simulink model "ExtraCredit"  (R2016a)
settings: Solver=VariableStepAuto  StartTime=0.0  StopTime=10.0  RelTol=1e-3
libraries: hdlsllib x17
(part 2 of 2)

== system ExtraCredit/Subsystem/Subsystem/MultiBlock44 ==
  SumIn : Inport
  Cin : Inport  Port=2
  B : Inport  Port=3
  A : Inport  Port=4
  AND : Logic  IconShape=distinctive  AllPortsSameDT=off  OutDataTypeStr=boolean
  AND1 : Logic  IconShape=distinctive  AllPortsSameDT=off  OutDataTypeStr=boolean
  AND2 : Logic  IconShape=distinctive  AllPortsSameDT=off  OutDataTypeStr=boolean
  "OR " : Logic  Operator=OR  IconShape=distinctive  AllPortsSameDT=off  OutDataTypeStr=boolean
  XOR : Logic  Operator=XOR  IconShape=distinctive  AllPortsSameDT=off  OutDataTypeStr=boolean
  XOR1 : Logic  Operator=XOR  IconShape=distinctive  AllPortsSameDT=off  OutDataTypeStr=boolean
  Sum : Outport
  Carry : Outport  Port=2
  wires:
  SumIn/1 -> XOR1/1, AND/1
  XOR1/1 -> AND1/1, XOR/1
  Cin/1 -> XOR/2, AND1/2
  XOR/1 -> Sum/1
  AND2/1 -> AND/2, XOR1/2
  "OR "/1 -> Carry/1
  AND1/1 -> "OR "/1
  AND/1 -> "OR "/2
  B/1 -> AND2/2
  A/1 -> AND2/1

== system ExtraCredit/Subsystem/Subsystem/MultiBlock45 ==
  SumIn : Inport
  Cin : Inport  Port=2
  B : Inport  Port=3
  A : Inport  Port=4
  AND : Logic  IconShape=distinctive  AllPortsSameDT=off  OutDataTypeStr=boolean
  AND1 : Logic  IconShape=distinctive  AllPortsSameDT=off  OutDataTypeStr=boolean
  AND2 : Logic  IconShape=distinctive  AllPortsSameDT=off  OutDataTypeStr=boolean
  "OR " : Logic  Operator=OR  IconShape=distinctive  AllPortsSameDT=off  OutDataTypeStr=boolean
  XOR : Logic  Operator=XOR  IconShape=distinctive  AllPortsSameDT=off  OutDataTypeStr=boolean
  XOR1 : Logic  Operator=XOR  IconShape=distinctive  AllPortsSameDT=off  OutDataTypeStr=boolean
  Sum : Outport
  Carry : Outport  Port=2
  wires:
  SumIn/1 -> XOR1/1, AND/1
  XOR1/1 -> AND1/1, XOR/1
  Cin/1 -> XOR/2, AND1/2
  XOR/1 -> Sum/1
  AND2/1 -> AND/2, XOR1/2
  "OR "/1 -> Carry/1
  AND1/1 -> "OR "/1
  AND/1 -> "OR "/2
  B/1 -> AND2/2
  A/1 -> AND2/1

== system ExtraCredit/Subsystem/Subsystem/MultiBlock46 ==
  SumIn : Inport
  Cin : Inport  Port=2
  B : Inport  Port=3
  A : Inport  Port=4
  AND : Logic  IconShape=distinctive  AllPortsSameDT=off  OutDataTypeStr=boolean
  AND1 : Logic  IconShape=distinctive  AllPortsSameDT=off  OutDataTypeStr=boolean
  AND2 : Logic  IconShape=distinctive  AllPortsSameDT=off  OutDataTypeStr=boolean
  "OR " : Logic  Operator=OR  IconShape=distinctive  AllPortsSameDT=off  OutDataTypeStr=boolean
  XOR : Logic  Operator=XOR  IconShape=distinctive  AllPortsSameDT=off  OutDataTypeStr=boolean
  XOR1 : Logic  Operator=XOR  IconShape=distinctive  AllPortsSameDT=off  OutDataTypeStr=boolean
  Sum : Outport
  Carry : Outport  Port=2
  wires:
  SumIn/1 -> XOR1/1, AND/1
  XOR1/1 -> AND1/1, XOR/1
  Cin/1 -> XOR/2, AND1/2
  XOR/1 -> Sum/1
  AND2/1 -> AND/2, XOR1/2
  "OR "/1 -> Carry/1
  AND1/1 -> "OR "/1
  AND/1 -> "OR "/2
  B/1 -> AND2/2
  A/1 -> AND2/1

== system ExtraCredit/Subsystem/Subsystem/MultiBlock47 ==
  SumIn : Inport
  Cin : Inport  Port=2
  B : Inport  Port=3
  A : Inport  Port=4
  AND : Logic  IconShape=distinctive  AllPortsSameDT=off  OutDataTypeStr=boolean
  AND1 : Logic  IconShape=distinctive  AllPortsSameDT=off  OutDataTypeStr=boolean
  AND2 : Logic  IconShape=distinctive  AllPortsSameDT=off  OutDataTypeStr=boolean
  "OR " : Logic  Operator=OR  IconShape=distinctive  AllPortsSameDT=off  OutDataTypeStr=boolean
  XOR : Logic  Operator=XOR  IconShape=distinctive  AllPortsSameDT=off  OutDataTypeStr=boolean
  XOR1 : Logic  Operator=XOR  IconShape=distinctive  AllPortsSameDT=off  OutDataTypeStr=boolean
  Sum : Outport
  Carry : Outport  Port=2
  wires:
  SumIn/1 -> XOR1/1, AND/1
  XOR1/1 -> AND1/1, XOR/1
  Cin/1 -> XOR/2, AND1/2
  XOR/1 -> Sum/1
  AND2/1 -> AND/2, XOR1/2
  "OR "/1 -> Carry/1
  AND1/1 -> "OR "/1
  AND/1 -> "OR "/2
  B/1 -> AND2/2
  A/1 -> AND2/1

== system ExtraCredit/Subsystem/Subsystem/MultiBlock48 ==
  SumIn : Inport
  Cin : Inport  Port=2
  B : Inport  Port=3
  A : Inport  Port=4
  AND : Logic  IconShape=distinctive  AllPortsSameDT=off  OutDataTypeStr=boolean
  AND1 : Logic  IconShape=distinctive  AllPortsSameDT=off  OutDataTypeStr=boolean
  AND2 : Logic  IconShape=distinctive  AllPortsSameDT=off  OutDataTypeStr=boolean
  "OR " : Logic  Operator=OR  IconShape=distinctive  AllPortsSameDT=off  OutDataTypeStr=boolean
  XOR : Logic  Operator=XOR  IconShape=distinctive  AllPortsSameDT=off  OutDataTypeStr=boolean
  XOR1 : Logic  Operator=XOR  IconShape=distinctive  AllPortsSameDT=off  OutDataTypeStr=boolean
  Sum : Outport
  Carry : Outport  Port=2
  wires:
  SumIn/1 -> XOR1/1, AND/1
  XOR1/1 -> AND1/1, XOR/1
  Cin/1 -> XOR/2, AND1/2
  XOR/1 -> Sum/1
  AND2/1 -> AND/2, XOR1/2
  "OR "/1 -> Carry/1
  AND1/1 -> "OR "/1
  AND/1 -> "OR "/2
  B/1 -> AND2/2
  A/1 -> AND2/1

== system ExtraCredit/Subsystem/Subsystem/MultiBlock49 ==
  SumIn : Inport
  Cin : Inport  Port=2
  B : Inport  Port=3
  A : Inport  Port=4
  AND : Logic  IconShape=distinctive  AllPortsSameDT=off  OutDataTypeStr=boolean
  AND1 : Logic  IconShape=distinctive  AllPortsSameDT=off  OutDataTypeStr=boolean
  AND2 : Logic  IconShape=distinctive  AllPortsSameDT=off  OutDataTypeStr=boolean
  "OR " : Logic  Operator=OR  IconShape=distinctive  AllPortsSameDT=off  OutDataTypeStr=boolean
  XOR : Logic  Operator=XOR  IconShape=distinctive  AllPortsSameDT=off  OutDataTypeStr=boolean
  XOR1 : Logic  Operator=XOR  IconShape=distinctive  AllPortsSameDT=off  OutDataTypeStr=boolean
  Sum : Outport
  Carry : Outport  Port=2
  wires:
  SumIn/1 -> XOR1/1, AND/1
  XOR1/1 -> AND1/1, XOR/1
  Cin/1 -> XOR/2, AND1/2
  XOR/1 -> Sum/1
  AND2/1 -> AND/2, XOR1/2
  "OR "/1 -> Carry/1
  AND1/1 -> "OR "/1
  AND/1 -> "OR "/2
  B/1 -> AND2/2
  A/1 -> AND2/1

== system ExtraCredit/Subsystem/Subsystem/MultiBlock5 ==
  SumIn : Inport
  Cin : Inport  Port=2
  B : Inport  Port=3
  A : Inport  Port=4
  AND : Logic  IconShape=distinctive  AllPortsSameDT=off  OutDataTypeStr=boolean
  AND1 : Logic  IconShape=distinctive  AllPortsSameDT=off  OutDataTypeStr=boolean
  AND2 : Logic  IconShape=distinctive  AllPortsSameDT=off  OutDataTypeStr=boolean
  "OR " : Logic  Operator=OR  IconShape=distinctive  AllPortsSameDT=off  OutDataTypeStr=boolean
  XOR : Logic  Operator=XOR  IconShape=distinctive  AllPortsSameDT=off  OutDataTypeStr=boolean
  XOR1 : Logic  Operator=XOR  IconShape=distinctive  AllPortsSameDT=off  OutDataTypeStr=boolean
  Sum : Outport
  Carry : Outport  Port=2
  wires:
  SumIn/1 -> XOR1/1, AND/1
  XOR1/1 -> AND1/1, XOR/1
  Cin/1 -> XOR/2, AND1/2
  XOR/1 -> Sum/1
  AND2/1 -> AND/2, XOR1/2
  "OR "/1 -> Carry/1
  AND1/1 -> "OR "/1
  AND/1 -> "OR "/2
  B/1 -> AND2/2
  A/1 -> AND2/1

== system ExtraCredit/Subsystem/Subsystem/MultiBlock50 ==
  SumIn : Inport
  Cin : Inport  Port=2
  B : Inport  Port=3
  A : Inport  Port=4
  AND : Logic  IconShape=distinctive  AllPortsSameDT=off  OutDataTypeStr=boolean
  AND1 : Logic  IconShape=distinctive  AllPortsSameDT=off  OutDataTypeStr=boolean
  AND2 : Logic  IconShape=distinctive  AllPortsSameDT=off  OutDataTypeStr=boolean
  "OR " : Logic  Operator=OR  IconShape=distinctive  AllPortsSameDT=off  OutDataTypeStr=boolean
  XOR : Logic  Operator=XOR  IconShape=distinctive  AllPortsSameDT=off  OutDataTypeStr=boolean
  XOR1 : Logic  Operator=XOR  IconShape=distinctive  AllPortsSameDT=off  OutDataTypeStr=boolean
  Sum : Outport
  Carry : Outport  Port=2
  wires:
  SumIn/1 -> XOR1/1, AND/1
  XOR1/1 -> AND1/1, XOR/1
  Cin/1 -> XOR/2, AND1/2
  XOR/1 -> Sum/1
  AND2/1 -> AND/2, XOR1/2
  "OR "/1 -> Carry/1
  AND1/1 -> "OR "/1
  AND/1 -> "OR "/2
  B/1 -> AND2/2
  A/1 -> AND2/1

== system ExtraCredit/Subsystem/Subsystem/MultiBlock51 ==
  SumIn : Inport
  Cin : Inport  Port=2
  B : Inport  Port=3
  A : Inport  Port=4
  AND : Logic  IconShape=distinctive  AllPortsSameDT=off  OutDataTypeStr=boolean
  AND1 : Logic  IconShape=distinctive  AllPortsSameDT=off  OutDataTypeStr=boolean
  AND2 : Logic  IconShape=distinctive  AllPortsSameDT=off  OutDataTypeStr=boolean
  "OR " : Logic  Operator=OR  IconShape=distinctive  AllPortsSameDT=off  OutDataTypeStr=boolean
  XOR : Logic  Operator=XOR  IconShape=distinctive  AllPortsSameDT=off  OutDataTypeStr=boolean
  XOR1 : Logic  Operator=XOR  IconShape=distinctive  AllPortsSameDT=off  OutDataTypeStr=boolean
  Sum : Outport
  Carry : Outport  Port=2
  wires:
  SumIn/1 -> XOR1/1, AND/1
  XOR1/1 -> AND1/1, XOR/1
  Cin/1 -> XOR/2, AND1/2
  XOR/1 -> Sum/1
  AND2/1 -> AND/2, XOR1/2
  "OR "/1 -> Carry/1
  AND1/1 -> "OR "/1
  AND/1 -> "OR "/2
  B/1 -> AND2/2
  A/1 -> AND2/1

== system ExtraCredit/Subsystem/Subsystem/MultiBlock52 ==
  SumIn : Inport
  Cin : Inport  Port=2
  B : Inport  Port=3
  A : Inport  Port=4
  AND : Logic  IconShape=distinctive  AllPortsSameDT=off  OutDataTypeStr=boolean
  AND1 : Logic  IconShape=distinctive  AllPortsSameDT=off  OutDataTypeStr=boolean
  AND2 : Logic  IconShape=distinctive  AllPortsSameDT=off  OutDataTypeStr=boolean
  "OR " : Logic  Operator=OR  IconShape=distinctive  AllPortsSameDT=off  OutDataTypeStr=boolean
  XOR : Logic  Operator=XOR  IconShape=distinctive  AllPortsSameDT=off  OutDataTypeStr=boolean
  XOR1 : Logic  Operator=XOR  IconShape=distinctive  AllPortsSameDT=off  OutDataTypeStr=boolean
  Sum : Outport
  Carry : Outport  Port=2
  wires:
  SumIn/1 -> XOR1/1, AND/1
  XOR1/1 -> AND1/1, XOR/1
  Cin/1 -> XOR/2, AND1/2
  XOR/1 -> Sum/1
  AND2/1 -> AND/2, XOR1/2
  "OR "/1 -> Carry/1
  AND1/1 -> "OR "/1
  AND/1 -> "OR "/2
  B/1 -> AND2/2
  A/1 -> AND2/1

== system ExtraCredit/Subsystem/Subsystem/MultiBlock53 ==
  SumIn : Inport
  Cin : Inport  Port=2
  B : Inport  Port=3
  A : Inport  Port=4
  AND : Logic  IconShape=distinctive  AllPortsSameDT=off  OutDataTypeStr=boolean
  AND1 : Logic  IconShape=distinctive  AllPortsSameDT=off  OutDataTypeStr=boolean
  AND2 : Logic  IconShape=distinctive  AllPortsSameDT=off  OutDataTypeStr=boolean
  "OR " : Logic  Operator=OR  IconShape=distinctive  AllPortsSameDT=off  OutDataTypeStr=boolean
  XOR : Logic  Operator=XOR  IconShape=distinctive  AllPortsSameDT=off  OutDataTypeStr=boolean
  XOR1 : Logic  Operator=XOR  IconShape=distinctive  AllPortsSameDT=off  OutDataTypeStr=boolean
  Sum : Outport
  Carry : Outport  Port=2
  wires:
  SumIn/1 -> XOR1/1, AND/1
  XOR1/1 -> AND1/1, XOR/1
  Cin/1 -> XOR/2, AND1/2
  XOR/1 -> Sum/1
  AND2/1 -> AND/2, XOR1/2
  "OR "/1 -> Carry/1
  AND1/1 -> "OR "/1
  AND/1 -> "OR "/2
  B/1 -> AND2/2
  A/1 -> AND2/1

== system ExtraCredit/Subsystem/Subsystem/MultiBlock54 ==
  SumIn : Inport
  Cin : Inport  Port=2
  B : Inport  Port=3
  A : Inport  Port=4
  AND : Logic  IconShape=distinctive  AllPortsSameDT=off  OutDataTypeStr=boolean
  AND1 : Logic  IconShape=distinctive  AllPortsSameDT=off  OutDataTypeStr=boolean
  AND2 : Logic  IconShape=distinctive  AllPortsSameDT=off  OutDataTypeStr=boolean
  "OR " : Logic  Operator=OR  IconShape=distinctive  AllPortsSameDT=off  OutDataTypeStr=boolean
  XOR : Logic  Operator=XOR  IconShape=distinctive  AllPortsSameDT=off  OutDataTypeStr=boolean
  XOR1 : Logic  Operator=XOR  IconShape=distinctive  AllPortsSameDT=off  OutDataTypeStr=boolean
  Sum : Outport
  Carry : Outport  Port=2
  wires:
  SumIn/1 -> XOR1/1, AND/1
  XOR1/1 -> AND1/1, XOR/1
  Cin/1 -> XOR/2, AND1/2
  XOR/1 -> Sum/1
  AND2/1 -> AND/2, XOR1/2
  "OR "/1 -> Carry/1
  AND1/1 -> "OR "/1
  AND/1 -> "OR "/2
  B/1 -> AND2/2
  A/1 -> AND2/1

== system ExtraCredit/Subsystem/Subsystem/MultiBlock55 ==
  SumIn : Inport
  Cin : Inport  Port=2
  B : Inport  Port=3
  A : Inport  Port=4
  AND : Logic  IconShape=distinctive  AllPortsSameDT=off  OutDataTypeStr=boolean
  AND1 : Logic  IconShape=distinctive  AllPortsSameDT=off  OutDataTypeStr=boolean
  AND2 : Logic  IconShape=distinctive  AllPortsSameDT=off  OutDataTypeStr=boolean
  "OR " : Logic  Operator=OR  IconShape=distinctive  AllPortsSameDT=off  OutDataTypeStr=boolean
  XOR : Logic  Operator=XOR  IconShape=distinctive  AllPortsSameDT=off  OutDataTypeStr=boolean
  XOR1 : Logic  Operator=XOR  IconShape=distinctive  AllPortsSameDT=off  OutDataTypeStr=boolean
  Sum : Outport
  Carry : Outport  Port=2
  wires:
  SumIn/1 -> XOR1/1, AND/1
  XOR1/1 -> AND1/1, XOR/1
  Cin/1 -> XOR/2, AND1/2
  XOR/1 -> Sum/1
  AND2/1 -> AND/2, XOR1/2
  "OR "/1 -> Carry/1
  AND1/1 -> "OR "/1
  AND/1 -> "OR "/2
  B/1 -> AND2/2
  A/1 -> AND2/1

== system ExtraCredit/Subsystem/Subsystem/MultiBlock56 ==
  SumIn : Inport
  Cin : Inport  Port=2
  B : Inport  Port=3
  A : Inport  Port=4
  AND : Logic  IconShape=distinctive  AllPortsSameDT=off  OutDataTypeStr=boolean
  AND1 : Logic  IconShape=distinctive  AllPortsSameDT=off  OutDataTypeStr=boolean
  AND2 : Logic  IconShape=distinctive  AllPortsSameDT=off  OutDataTypeStr=boolean
  "OR " : Logic  Operator=OR  IconShape=distinctive  AllPortsSameDT=off  OutDataTypeStr=boolean
  XOR : Logic  Operator=XOR  IconShape=distinctive  AllPortsSameDT=off  OutDataTypeStr=boolean
  XOR1 : Logic  Operator=XOR  IconShape=distinctive  AllPortsSameDT=off  OutDataTypeStr=boolean
  Sum : Outport
  Carry : Outport  Port=2
  wires:
  SumIn/1 -> XOR1/1, AND/1
  XOR1/1 -> AND1/1, XOR/1
  Cin/1 -> XOR/2, AND1/2
  XOR/1 -> Sum/1
  AND2/1 -> AND/2, XOR1/2
  "OR "/1 -> Carry/1
  AND1/1 -> "OR "/1
  AND/1 -> "OR "/2
  B/1 -> AND2/2
  A/1 -> AND2/1

== system ExtraCredit/Subsystem/Subsystem/MultiBlock57 ==
  SumIn : Inport
  Cin : Inport  Port=2
  B : Inport  Port=3
  A : Inport  Port=4
  AND : Logic  IconShape=distinctive  AllPortsSameDT=off  OutDataTypeStr=boolean
  AND1 : Logic  IconShape=distinctive  AllPortsSameDT=off  OutDataTypeStr=boolean
  AND2 : Logic  IconShape=distinctive  AllPortsSameDT=off  OutDataTypeStr=boolean
  "OR " : Logic  Operator=OR  IconShape=distinctive  AllPortsSameDT=off  OutDataTypeStr=boolean
  XOR : Logic  Operator=XOR  IconShape=distinctive  AllPortsSameDT=off  OutDataTypeStr=boolean
  XOR1 : Logic  Operator=XOR  IconShape=distinctive  AllPortsSameDT=off  OutDataTypeStr=boolean
  Sum : Outport
  Carry : Outport  Port=2
  wires:
  SumIn/1 -> XOR1/1, AND/1
  XOR1/1 -> AND1/1, XOR/1
  Cin/1 -> XOR/2, AND1/2
  XOR/1 -> Sum/1
  AND2/1 -> AND/2, XOR1/2
  "OR "/1 -> Carry/1
  AND1/1 -> "OR "/1
  AND/1 -> "OR "/2
  B/1 -> AND2/2
  A/1 -> AND2/1

== system ExtraCredit/Subsystem/Subsystem/MultiBlock58 ==
  SumIn : Inport
  Cin : Inport  Port=2
  B : Inport  Port=3
  A : Inport  Port=4
  AND : Logic  IconShape=distinctive  AllPortsSameDT=off  OutDataTypeStr=boolean
  AND1 : Logic  IconShape=distinctive  AllPortsSameDT=off  OutDataTypeStr=boolean
  AND2 : Logic  IconShape=distinctive  AllPortsSameDT=off  OutDataTypeStr=boolean
  "OR " : Logic  Operator=OR  IconShape=distinctive  AllPortsSameDT=off  OutDataTypeStr=boolean
  XOR : Logic  Operator=XOR  IconShape=distinctive  AllPortsSameDT=off  OutDataTypeStr=boolean
  XOR1 : Logic  Operator=XOR  IconShape=distinctive  AllPortsSameDT=off  OutDataTypeStr=boolean
  Sum : Outport
  Carry : Outport  Port=2
  wires:
  SumIn/1 -> XOR1/1, AND/1
  XOR1/1 -> AND1/1, XOR/1
  Cin/1 -> XOR/2, AND1/2
  XOR/1 -> Sum/1
  AND2/1 -> AND/2, XOR1/2
  "OR "/1 -> Carry/1
  AND1/1 -> "OR "/1
  AND/1 -> "OR "/2
  B/1 -> AND2/2
  A/1 -> AND2/1

== system ExtraCredit/Subsystem/Subsystem/MultiBlock59 ==
  SumIn : Inport
  Cin : Inport  Port=2
  B : Inport  Port=3
  A : Inport  Port=4
  AND : Logic  IconShape=distinctive  AllPortsSameDT=off  OutDataTypeStr=boolean
  AND1 : Logic  IconShape=distinctive  AllPortsSameDT=off  OutDataTypeStr=boolean
  AND2 : Logic  IconShape=distinctive  AllPortsSameDT=off  OutDataTypeStr=boolean
  "OR " : Logic  Operator=OR  IconShape=distinctive  AllPortsSameDT=off  OutDataTypeStr=boolean
  XOR : Logic  Operator=XOR  IconShape=distinctive  AllPortsSameDT=off  OutDataTypeStr=boolean
  XOR1 : Logic  Operator=XOR  IconShape=distinctive  AllPortsSameDT=off  OutDataTypeStr=boolean
  Sum : Outport
  Carry : Outport  Port=2
  wires:
  SumIn/1 -> XOR1/1, AND/1
  XOR1/1 -> AND1/1, XOR/1
  Cin/1 -> XOR/2, AND1/2
  XOR/1 -> Sum/1
  AND2/1 -> AND/2, XOR1/2
  "OR "/1 -> Carry/1
  AND1/1 -> "OR "/1
  AND/1 -> "OR "/2
  B/1 -> AND2/2
  A/1 -> AND2/1

== system ExtraCredit/Subsystem/Subsystem/MultiBlock6 ==
  SumIn : Inport
  Cin : Inport  Port=2
  B : Inport  Port=3
  A : Inport  Port=4
  AND : Logic  IconShape=distinctive  AllPortsSameDT=off  OutDataTypeStr=boolean
  AND1 : Logic  IconShape=distinctive  AllPortsSameDT=off  OutDataTypeStr=boolean
  AND2 : Logic  IconShape=distinctive  AllPortsSameDT=off  OutDataTypeStr=boolean
  "OR " : Logic  Operator=OR  IconShape=distinctive  AllPortsSameDT=off  OutDataTypeStr=boolean
  XOR : Logic  Operator=XOR  IconShape=distinctive  AllPortsSameDT=off  OutDataTypeStr=boolean
  XOR1 : Logic  Operator=XOR  IconShape=distinctive  AllPortsSameDT=off  OutDataTypeStr=boolean
  Sum : Outport
  Carry : Outport  Port=2
  wires:
  SumIn/1 -> XOR1/1, AND/1
  XOR1/1 -> AND1/1, XOR/1
  Cin/1 -> XOR/2, AND1/2
  XOR/1 -> Sum/1
  AND2/1 -> AND/2, XOR1/2
  "OR "/1 -> Carry/1
  AND1/1 -> "OR "/1
  AND/1 -> "OR "/2
  B/1 -> AND2/2
  A/1 -> AND2/1

== system ExtraCredit/Subsystem/Subsystem/MultiBlock60 ==
  SumIn : Inport
  Cin : Inport  Port=2
  B : Inport  Port=3
  A : Inport  Port=4
  AND : Logic  IconShape=distinctive  AllPortsSameDT=off  OutDataTypeStr=boolean
  AND1 : Logic  IconShape=distinctive  AllPortsSameDT=off  OutDataTypeStr=boolean
  AND2 : Logic  IconShape=distinctive  AllPortsSameDT=off  OutDataTypeStr=boolean
  "OR " : Logic  Operator=OR  IconShape=distinctive  AllPortsSameDT=off  OutDataTypeStr=boolean
  XOR : Logic  Operator=XOR  IconShape=distinctive  AllPortsSameDT=off  OutDataTypeStr=boolean
  XOR1 : Logic  Operator=XOR  IconShape=distinctive  AllPortsSameDT=off  OutDataTypeStr=boolean
  Sum : Outport
  Carry : Outport  Port=2
  wires:
  SumIn/1 -> XOR1/1, AND/1
  XOR1/1 -> AND1/1, XOR/1
  Cin/1 -> XOR/2, AND1/2
  XOR/1 -> Sum/1
  AND2/1 -> AND/2, XOR1/2
  "OR "/1 -> Carry/1
  AND1/1 -> "OR "/1
  AND/1 -> "OR "/2
  B/1 -> AND2/2
  A/1 -> AND2/1

== system ExtraCredit/Subsystem/Subsystem/MultiBlock61 ==
  SumIn : Inport
  Cin : Inport  Port=2
  B : Inport  Port=3
  A : Inport  Port=4
  AND : Logic  IconShape=distinctive  AllPortsSameDT=off  OutDataTypeStr=boolean
  AND1 : Logic  IconShape=distinctive  AllPortsSameDT=off  OutDataTypeStr=boolean
  AND2 : Logic  IconShape=distinctive  AllPortsSameDT=off  OutDataTypeStr=boolean
  "OR " : Logic  Operator=OR  IconShape=distinctive  AllPortsSameDT=off  OutDataTypeStr=boolean
  XOR : Logic  Operator=XOR  IconShape=distinctive  AllPortsSameDT=off  OutDataTypeStr=boolean
  XOR1 : Logic  Operator=XOR  IconShape=distinctive  AllPortsSameDT=off  OutDataTypeStr=boolean
  Sum : Outport
  Carry : Outport  Port=2
  wires:
  SumIn/1 -> XOR1/1, AND/1
  XOR1/1 -> AND1/1, XOR/1
  Cin/1 -> XOR/2, AND1/2
  XOR/1 -> Sum/1
  AND2/1 -> AND/2, XOR1/2
  "OR "/1 -> Carry/1
  AND1/1 -> "OR "/1
  AND/1 -> "OR "/2
  B/1 -> AND2/2
  A/1 -> AND2/1

== system ExtraCredit/Subsystem/Subsystem/MultiBlock62 ==
  SumIn : Inport
  Cin : Inport  Port=2
  B : Inport  Port=3
  A : Inport  Port=4
  AND : Logic  IconShape=distinctive  AllPortsSameDT=off  OutDataTypeStr=boolean
  AND1 : Logic  IconShape=distinctive  AllPortsSameDT=off  OutDataTypeStr=boolean
  AND2 : Logic  IconShape=distinctive  AllPortsSameDT=off  OutDataTypeStr=boolean
  "OR " : Logic  Operator=OR  IconShape=distinctive  AllPortsSameDT=off  OutDataTypeStr=boolean
  XOR : Logic  Operator=XOR  IconShape=distinctive  AllPortsSameDT=off  OutDataTypeStr=boolean
  XOR1 : Logic  Operator=XOR  IconShape=distinctive  AllPortsSameDT=off  OutDataTypeStr=boolean
  Sum : Outport
  Carry : Outport  Port=2
  wires:
  SumIn/1 -> XOR1/1, AND/1
  XOR1/1 -> AND1/1, XOR/1
  Cin/1 -> XOR/2, AND1/2
  XOR/1 -> Sum/1
  AND2/1 -> AND/2, XOR1/2
  "OR "/1 -> Carry/1
  AND1/1 -> "OR "/1
  AND/1 -> "OR "/2
  B/1 -> AND2/2
  A/1 -> AND2/1

== system ExtraCredit/Subsystem/Subsystem/MultiBlock63 ==
  SumIn : Inport
  Cin : Inport  Port=2
  B : Inport  Port=3
  A : Inport  Port=4
  AND : Logic  IconShape=distinctive  AllPortsSameDT=off  OutDataTypeStr=boolean
  AND1 : Logic  IconShape=distinctive  AllPortsSameDT=off  OutDataTypeStr=boolean
  AND2 : Logic  IconShape=distinctive  AllPortsSameDT=off  OutDataTypeStr=boolean
  "OR " : Logic  Operator=OR  IconShape=distinctive  AllPortsSameDT=off  OutDataTypeStr=boolean
  XOR : Logic  Operator=XOR  IconShape=distinctive  AllPortsSameDT=off  OutDataTypeStr=boolean
  XOR1 : Logic  Operator=XOR  IconShape=distinctive  AllPortsSameDT=off  OutDataTypeStr=boolean
  Sum : Outport
  Carry : Outport  Port=2
  wires:
  SumIn/1 -> XOR1/1, AND/1
  XOR1/1 -> AND1/1, XOR/1
  Cin/1 -> XOR/2, AND1/2
  XOR/1 -> Sum/1
  AND2/1 -> AND/2, XOR1/2
  "OR "/1 -> Carry/1
  AND1/1 -> "OR "/1
  AND/1 -> "OR "/2
  B/1 -> AND2/2
  A/1 -> AND2/1

== system ExtraCredit/Subsystem/Subsystem/MultiBlock7 ==
  SumIn : Inport
  Cin : Inport  Port=2
  B : Inport  Port=3
  A : Inport  Port=4
  AND : Logic  IconShape=distinctive  AllPortsSameDT=off  OutDataTypeStr=boolean
  AND1 : Logic  IconShape=distinctive  AllPortsSameDT=off  OutDataTypeStr=boolean
  AND2 : Logic  IconShape=distinctive  AllPortsSameDT=off  OutDataTypeStr=boolean
  "OR " : Logic  Operator=OR  IconShape=distinctive  AllPortsSameDT=off  OutDataTypeStr=boolean
  XOR : Logic  Operator=XOR  IconShape=distinctive  AllPortsSameDT=off  OutDataTypeStr=boolean
  XOR1 : Logic  Operator=XOR  IconShape=distinctive  AllPortsSameDT=off  OutDataTypeStr=boolean
  Sum : Outport
  Carry : Outport  Port=2
  wires:
  SumIn/1 -> XOR1/1, AND/1
  XOR1/1 -> AND1/1, XOR/1
  Cin/1 -> XOR/2, AND1/2
  XOR/1 -> Sum/1
  AND2/1 -> AND/2, XOR1/2
  "OR "/1 -> Carry/1
  AND1/1 -> "OR "/1
  AND/1 -> "OR "/2
  B/1 -> AND2/2
  A/1 -> AND2/1

== system ExtraCredit/Subsystem/Subsystem/MultiBlock8 ==
  SumIn : Inport
  Cin : Inport  Port=2
  B : Inport  Port=3
  A : Inport  Port=4
  AND : Logic  IconShape=distinctive  AllPortsSameDT=off  OutDataTypeStr=boolean
  AND1 : Logic  IconShape=distinctive  AllPortsSameDT=off  OutDataTypeStr=boolean
  AND2 : Logic  IconShape=distinctive  AllPortsSameDT=off  OutDataTypeStr=boolean
  "OR " : Logic  Operator=OR  IconShape=distinctive  AllPortsSameDT=off  OutDataTypeStr=boolean
  XOR : Logic  Operator=XOR  IconShape=distinctive  AllPortsSameDT=off  OutDataTypeStr=boolean
  XOR1 : Logic  Operator=XOR  IconShape=distinctive  AllPortsSameDT=off  OutDataTypeStr=boolean
  Sum : Outport
  Carry : Outport  Port=2
  wires:
  SumIn/1 -> XOR1/1, AND/1
  XOR1/1 -> AND1/1, XOR/1
  Cin/1 -> XOR/2, AND1/2
  XOR/1 -> Sum/1
  AND2/1 -> AND/2, XOR1/2
  "OR "/1 -> Carry/1
  AND1/1 -> "OR "/1
  AND/1 -> "OR "/2
  B/1 -> AND2/2
  A/1 -> AND2/1

== system ExtraCredit/Subsystem/Subsystem/MultiBlock9 ==
  SumIn : Inport
  Cin : Inport  Port=2
  B : Inport  Port=3
  A : Inport  Port=4
  AND : Logic  IconShape=distinctive  AllPortsSameDT=off  OutDataTypeStr=boolean
  AND1 : Logic  IconShape=distinctive  AllPortsSameDT=off  OutDataTypeStr=boolean
  AND2 : Logic  IconShape=distinctive  AllPortsSameDT=off  OutDataTypeStr=boolean
  "OR " : Logic  Operator=OR  IconShape=distinctive  AllPortsSameDT=off  OutDataTypeStr=boolean
  XOR : Logic  Operator=XOR  IconShape=distinctive  AllPortsSameDT=off  OutDataTypeStr=boolean
  XOR1 : Logic  Operator=XOR  IconShape=distinctive  AllPortsSameDT=off  OutDataTypeStr=boolean
  Sum : Outport
  Carry : Outport  Port=2
  wires:
  SumIn/1 -> XOR1/1, AND/1
  XOR1/1 -> AND1/1, XOR/1
  Cin/1 -> XOR/2, AND1/2
  XOR/1 -> Sum/1
  AND2/1 -> AND/2, XOR1/2
  "OR "/1 -> Carry/1
  AND1/1 -> "OR "/1
  AND/1 -> "OR "/2
  B/1 -> AND2/2
  A/1 -> AND2/1

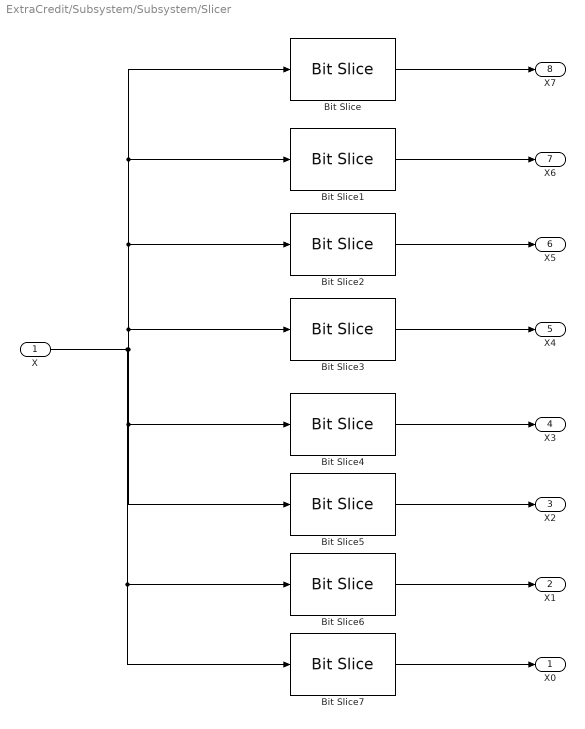
== system ExtraCredit/Subsystem/Subsystem/Slicer ==
  X : Inport  OutDataTypeStr=int8  SampleTime=1
  Bit Slice : hdlsllib/HDL Operations/Bit Slice  lidx=7  ridx=7
  Bit Slice1 : hdlsllib/HDL Operations/Bit Slice  lidx=6  ridx=6
  Bit Slice2 : hdlsllib/HDL Operations/Bit Slice  lidx=5  ridx=5
  Bit Slice3 : hdlsllib/HDL Operations/Bit Slice  lidx=4  ridx=4
  Bit Slice4 : hdlsllib/HDL Operations/Bit Slice  lidx=3  ridx=3
  Bit Slice5 : hdlsllib/HDL Operations/Bit Slice  lidx=2  ridx=2
  Bit Slice6 : hdlsllib/HDL Operations/Bit Slice  lidx=1  ridx=1
  Bit Slice7 : hdlsllib/HDL Operations/Bit Slice  lidx=0  ridx=0
  X0 : Outport
  X1 : Outport  Port=2
  X2 : Outport  Port=3
  X3 : Outport  Port=4
  X4 : Outport  Port=5
  X5 : Outport  Port=6
  X6 : Outport  Port=7
  X7 : Outport  Port=8
  wires:
  Bit Slice7/1 -> X0/1
  Bit Slice6/1 -> X1/1
  Bit Slice3/1 -> X4/1
  Bit Slice/1 -> X7/1
  Bit Slice5/1 -> X2/1
  Bit Slice4/1 -> X3/1
  Bit Slice1/1 -> X6/1
  Bit Slice2/1 -> X5/1
  X/1 -> Bit Slice7/1, Bit Slice6/1, Bit Slice3/1, Bit Slice/1, Bit Slice1/1, Bit Slice2/1, Bit Slice4/1, Bit Slice5/1

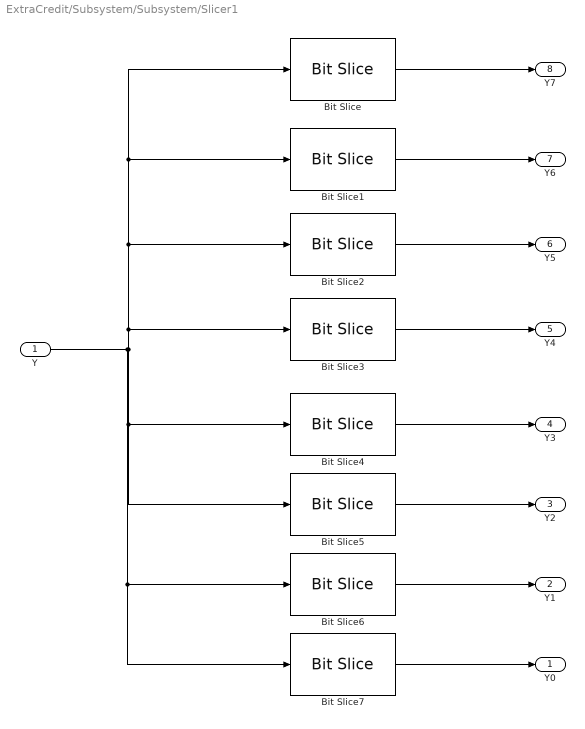
== system ExtraCredit/Subsystem/Subsystem/Slicer1 ==
  Y : Inport  OutDataTypeStr=int8  SampleTime=1
  Bit Slice : hdlsllib/HDL Operations/Bit Slice  lidx=7  ridx=7
  Bit Slice1 : hdlsllib/HDL Operations/Bit Slice  lidx=6  ridx=6
  Bit Slice2 : hdlsllib/HDL Operations/Bit Slice  lidx=5  ridx=5
  Bit Slice3 : hdlsllib/HDL Operations/Bit Slice  lidx=4  ridx=4
  Bit Slice4 : hdlsllib/HDL Operations/Bit Slice  lidx=3  ridx=3
  Bit Slice5 : hdlsllib/HDL Operations/Bit Slice  lidx=2  ridx=2
  Bit Slice6 : hdlsllib/HDL Operations/Bit Slice  lidx=1  ridx=1
  Bit Slice7 : hdlsllib/HDL Operations/Bit Slice  lidx=0  ridx=0
  Y0 : Outport
  Y1 : Outport  Port=2
  Y2 : Outport  Port=3
  Y3 : Outport  Port=4
  Y4 : Outport  Port=5
  Y5 : Outport  Port=6
  Y6 : Outport  Port=7
  Y7 : Outport  Port=8
  wires:
  Bit Slice7/1 -> Y0/1
  Bit Slice6/1 -> Y1/1
  Bit Slice3/1 -> Y4/1
  Bit Slice/1 -> Y7/1
  Bit Slice5/1 -> Y2/1
  Bit Slice4/1 -> Y3/1
  Bit Slice1/1 -> Y6/1
  Bit Slice2/1 -> Y5/1
  Y/1 -> Bit Slice7/1, Bit Slice6/1, Bit Slice3/1, Bit Slice/1, Bit Slice1/1, Bit Slice2/1, Bit Slice4/1, Bit Slice5/1
